simulink model "bungee"  (R2022b)
settings: Solver=VariableStepAuto  StartTime=0.0  StopTime=50  RelTol=1e-3  EnableMultiTasking=on
PreLoadFcn:
  | % Execute script to load parameters
  | bungeeParams;
values from neighbouring files (symbols this model uses):
  A = pi*d^2/4    (= 0.00441786466911)    [ballParams.m]    (also in bungeeParams.m = 0.5)
  CD = 0.3    [ballParams.m]    (also in bmwParams.m = 0.4; bungeeParams.m = 0.6)
  g = 9.81    [ballParams.m]    (also in bungeeParams.m)
  k = 25    [bungeeParams.m]
  L = 20    [bungeeParams.m]
  m = 0.145    [ballParams.m]    (also in bmwParams.m = 104.2; bungeeParams.m = 90)
  rho = 1.2    [ballParams.m]    (also in bmwParams.m = 0.002377; bungeeParams.m)
  x0 = 80    [bungeeParams.m]
settings Model: Creator=nicholas  LastModifiedBy=bensweet
settings SolverCC: AlgebraicLoopSolver=TrustRegion
settings DataIOCC: SaveFormat=Array  SaveState=on  ReturnWorkspaceOutputs=off  SignalLoggingName=sigsOut
settings OptimizationCC: BlockReduction=off  BooleanDataType=off  ExpressionDepthLimit=2147483647  InitFltsAndDblsToZero=on  LifeSpan=inf
settings DebuggingCC: CheckExecutionContextPreStartOutputMsg=on  UnconnectedInputMsg=warning  UnconnectedOutputMsg=warning  UnconnectedLineMsg=warning  PregeneratedLibrarySubsystemCodeDiagnostic=none  SFMachineParentedDataDiag=warning
settings HardwareCC: ProdBitPerPointer=32  ProdBitPerSizeT=32  ProdBitPerPtrDiffT=32  ProdLargestAtomicFloat=None  ProdIntDivRoundTo=Undefined  ProdEndianess=Unspecified  ProdWordSize=32  ProdHWDeviceType=32-bit Generic  TargetUnknown=on
settings ModelReferenceCC: EnableRefExpFcnMdlSchedulingChecks=on  PropagateSignalLabelsOutOfModel=off
settings SFSimCC: SimUseLocalCustomCode=off
settings RTWCC: RTWUseLocalCustomCode=off  DLArmComputeVersion=19.05
settings CodeAppCC: StateflowObjectComments=on
settings GRTTargetCC: TargetFcnLib=ansi_tfl_tmw.mat  TargetLangStandard=C89/C90 (ANSI)  CombineOutputUpdateFcns=off  GRTInterface=on
settings ConfigComp: CovMetricSettings=dw  CovSaveCumulativeToWorkspaceVar=on  CovSaveSingleToWorkspaceVar=on  CovExternalEMLEnable=off  CovSFcnEnable=off

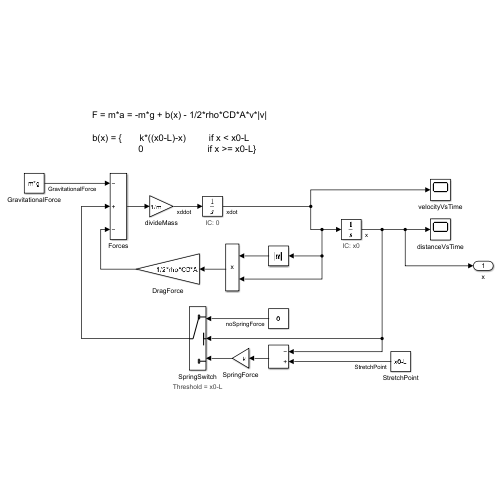
[thumbnail: Simulink's stored preview of the top-level diagram]
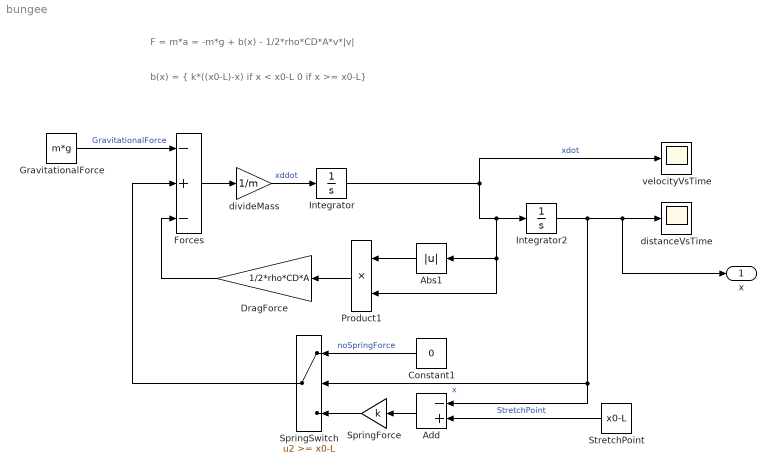
== system bungee ==
  note: b(x) = { k*((x0-L)-x) if x < x0-L
      | 0 if x >= x0-L}
  note: F = m*a = -m*g + b(x) - 1/2*rho*CD*A*v*|v|
  Abs1 : Abs  SaturateOnIntegerOverflow=off
  Add : Sum  Inputs=-+
  Constant1 : Constant  Value=0
  DragForce : Gain  Gain=1/2*rho*CD*A
  Forces : Sum  Inputs=-+-  InputSameDT=on  SaturateOnIntegerOverflow=on  OutDataTypeStr=Inherit: Same as first input
  GravitationalForce : Constant  Value=m*g
  Integrator : Integrator
      settings: AttributesFormatString=IC: %<InitialCondition>
  Integrator2 : Integrator  InitialCondition=x0
      settings: AttributesFormatString=IC: %<InitialCondition>
  Product1 : Product  RndMeth=Zero
  SpringForce : Gain  Gain=k  SaturateOnIntegerOverflow=on  OutDataTypeStr=Inherit: Same as input  ParamDataTypeStr=Inherit: Same as input
  SpringSwitch : Switch  Threshold=x0-L
      settings: AttributesFormatString=Threshold = %<Threshold>
  StretchPoint : Constant  Value=x0-L
  distanceVsTime : Scope
  divideMass : Gain  Gain=1/m  SaturateOnIntegerOverflow=on  OutDataTypeStr=Inherit: Same as input  ParamDataTypeStr=Inherit: Same as input
  velocityVsTime : Scope
  x : Outport  VectorParamsAs1DForOutWhenUnconnected=off
  wires:
  SpringSwitch/1 -> Forces/2
  Add/1 -> SpringForce/1
  divideMass/1 -> Integrator/1  "xddot"
  Integrator2/1 -> x/1, distanceVsTime/1, Add/1, SpringSwitch/2  "x"
  Abs1/1 -> Product1/1
  Constant1/1 -> SpringSwitch/1  "noSpringForce"
  SpringForce/1 -> SpringSwitch/3
  DragForce/1 -> Forces/3
  Integrator/1 -> Integrator2/1, Abs1/1, Product1/2, velocityVsTime/1  "xdot"
  Forces/1 -> divideMass/1
  Product1/1 -> DragForce/1
  GravitationalForce/1 -> Forces/1  "GravitationalForce"
  StretchPoint/1 -> Add/2  "StretchPoint"
